simulink model "xpcUEIMasterSlaveFrame"  (Simulink 6.0)
settings: Solver=FixedStepDiscrete  SolverMode=SingleTasking  StartTime=0.0  StopTime=inf  RelTol=1e-3
undefined symbols (not defined in the file or in its folder): MF, MFS, PD2
libraries: xpclib x6, dspsigattribs x4
settings Model: Creator=gweast  LastModifiedBy=ekbas  ExtModeArmWhenConnect=off  BufferReuse=off  ProdHWDeviceType=Specified
settings DataIOCC: SignalLoggingName=sigsOut
settings OptimizationCC: BooleanDataType=off  InlineInvariantSignals=off  OptimizeBlockIOStorage=off  BufferReuse=off  EnforceIntegerDowncast=off  FoldNonRolledExpr=off  LocalBlockOutputs=off  MultiInstanced=off
settings FormatCC: IgnoreBidirectionalLines=off
settings HardwareCC: ProdHWDeviceType=Specified
settings RTWCC: SystemTargetFile=xpctarget.tlc  TemplateMakefile=xpc_default_tmf  ProcessScript=xpctarget_make_rtw_hook
settings CodeAppCC: SimulinkBlockComments=off
settings xpcTargetCC: TargetFcnLib=iso_c_tmw.mat

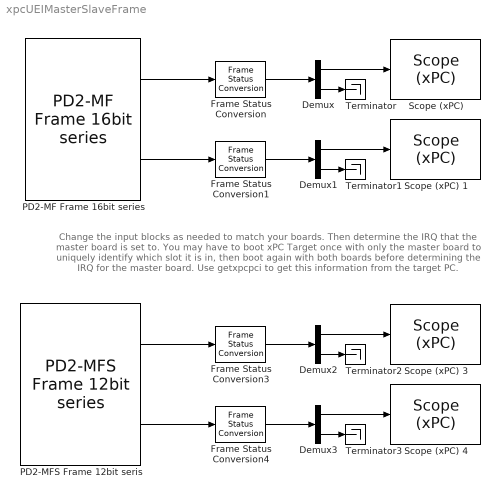
== system xpcUEIMasterSlaveFrame ==
  note: Change the input blocks as needed to match your boards.  Then determine
      | the IRQ that the master board is set to.  You may have to boot xPC Target
      | once with only the master board to uniquely identify which slot it is in, then
      | boot again with both boards before determining the IRQ for the master board.
      | Use getxpcpci to get this information from the target PC.
  Demux{,1..3} (4 alike) : Demux  Outputs=[1 -1]
  Frame Status Conversion{,1,3..4} (4 alike) : dspsigattribs/Frame Status Conversion  growRefPort=off  outframe=Sample-based
  "PD2-MF Frame 16bit series " : xpclib/A//D Frame/UEI/PD2-MF Frame 16bit series   boardtypein=PD2-MF-16-333/16H  channel=[1 2]  gain=[1]  mux=[0]  range=+- 10 Volts  sediff=Single Ended  framesize=32  outfmt=Frame (Signal Processing blockset needed)  clsource=Internal  scantime=-1  frametime=0.001  sampletime=off  slave=off  freq=-1  burst=32  pcislot=-1
  "PD2-MFS Frame 12bit seris " : xpclib/A//D Frame/UEI/PD2-MFS Frame 12bit series   boardtypein=PD2-MFS-8-1M/12H  channel=[1 2]  gain=[1]  mux=[0]  range=+- 10 Volts  framesize=32  outfmt=Frame (Signal Processing blockset needed)  clsource=Internal  scantime=-1  frametime=0.001  sampletime=off  slave=off  freq=-1  burst=32  pcislot=-1
  "Scope (xPC) " : xpclib/Misc./Scope (xPC)   scopeno=1  scopetype=Target  autostart=on  viewmode=Graphical redraw  formatstr='%15.6f'  grid=on  ylimits=[0,0]  nosamples=500  noprepostsamples=0  interleave=1  triggermode=FreeRun  triggersignal=1  triggerlevel=0.0  triggerslope=Either  triggerscope=1  triggersample=0  filename=data.dat  mode=Lazy  writesize=512  autorestart=off
  Scope (xPC) 1 : xpclib/Misc./Scope (xPC)   scopeno=2  scopetype=Target  autostart=on  viewmode=Graphical redraw  formatstr='%15.6f'  grid=on  ylimits=[0,0]  nosamples=500  noprepostsamples=0  interleave=1  triggermode=FreeRun  triggersignal=1  triggerlevel=0.0  triggerslope=Either  triggerscope=1  triggersample=0  filename=data.dat  mode=Lazy  writesize=512  autorestart=off
  Scope (xPC) 3 : xpclib/Misc./Scope (xPC)   scopeno=4  scopetype=Target  autostart=on  viewmode=Graphical redraw  formatstr='%15.6f'  grid=on  ylimits=[0,0]  nosamples=500  noprepostsamples=0  interleave=1  triggermode=FreeRun  triggersignal=1  triggerlevel=0.0  triggerslope=Either  triggerscope=1  triggersample=0  filename=data.dat  mode=Lazy  writesize=512  autorestart=off
  Scope (xPC) 4 : xpclib/Misc./Scope (xPC)   scopeno=5  scopetype=Target  autostart=on  viewmode=Graphical redraw  formatstr='%15.6f'  grid=on  ylimits=[0,0]  nosamples=500  noprepostsamples=0  interleave=1  triggermode=FreeRun  triggersignal=1  triggerlevel=0.0  triggerslope=Either  triggerscope=1  triggersample=0  filename=data.dat  mode=Lazy  writesize=512  autorestart=off
  Terminator{,1..3} (4 alike) : Terminator
  wires:
  "PD2-MF Frame 16bit series "/1 -> Frame Status Conversion/1
  "PD2-MF Frame 16bit series "/2 -> Frame Status Conversion1/1
  "PD2-MFS Frame 12bit seris "/1 -> Frame Status Conversion3/1
  "PD2-MFS Frame 12bit seris "/2 -> Frame Status Conversion4/1
  Frame Status Conversion/1 -> Demux/1
  Demux/1 -> "Scope (xPC) "/1
  Demux/2 -> Terminator/1
  Frame Status Conversion1/1 -> Demux1/1
  Demux1/1 -> Scope (xPC) 1/1
  Demux1/2 -> Terminator1/1
  Frame Status Conversion3/1 -> Demux2/1
  Demux2/1 -> Scope (xPC) 3/1
  Demux2/2 -> Terminator2/1
  Demux3/1 -> Scope (xPC) 4/1
  Demux3/2 -> Terminator3/1
  Frame Status Conversion4/1 -> Demux3/1
